simulink model "inv_rot_pen_simscape_vs_analytical_vs_detailed_sim_vs_real"  (R2025b)
settings: Solver=FixedStepAuto  StartTime=0.0  StopTime=4  FixedStep=Ts_fast  MaxStep=1e-3  RelTol=1e-3
values from neighbouring files (symbols this model uses):
  cfg = loaded.cfg    [continueFurutaMatlabSwingupTraining.m]    (also in evaluateFurutaController.m = makeFurutaConfig(); evaluateFurutaMatlabSwingupAgent.m = makeFurutaMatlabSwingupTD3Config(); finalizeFurutaDirectTD3Run.m = normalizeRunConfig(cfg, runDir); initFurutaSldrtHardwareWorkspace.m = makeFurutaMathWorksStyleWideTD3Config())
  i_max = 4    [initFurutaModelWorkspace.m]
  Kp_i = db2mag(options.CurrentControllerKpDb)    [initFurutaModelWorkspace.m]    (also in initFurutaSldrtHardwareWorkspace.m = 2.5)
  omega0 = options.InitialOmega    [initFurutaModelWorkspace.m]
  param = get_parameter()    [initFurutaModelWorkspace.m]
  s = zpk("s")    [initFurutaModelWorkspace.m]    (also in initFurutaSldrtHardwareWorkspace.m)
  theta0 = options.InitialTheta    [initFurutaModelWorkspace.m]
  Tn_i = param.L / param.R    [initFurutaModelWorkspace.m]    (also in initFurutaSldrtHardwareWorkspace.m = 0.000286849073257)
  Ts_fast = cfg.Model.HardwareFastSampleTime    [initFurutaSldrtHardwareWorkspace.m]
undefined symbols (not defined in the file or in its folder): currentBias_A, currentNoiseStd_A, DiscIntNeverNeededParam, G_diff_theta1_ss, G_diff_theta2, G_diff_theta2_ss, G_encoder_notch_d_ss, X, Y, Z
libraries: sm_lib x57, nesl_utility x18, cstblocks x13
(part 1 of 3)
settings Model: Creator=pichim  LastModifiedBy=abuj

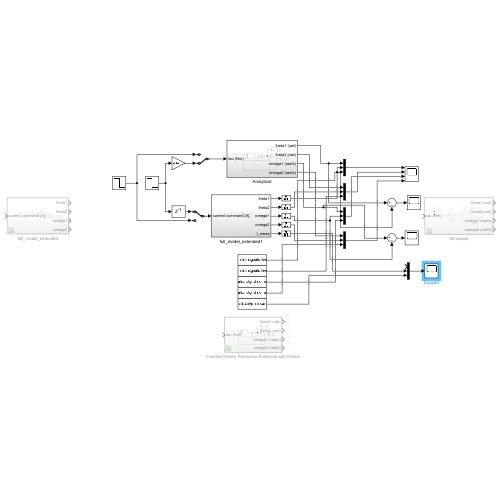
[thumbnail: Simulink's stored preview of the top-level diagram]
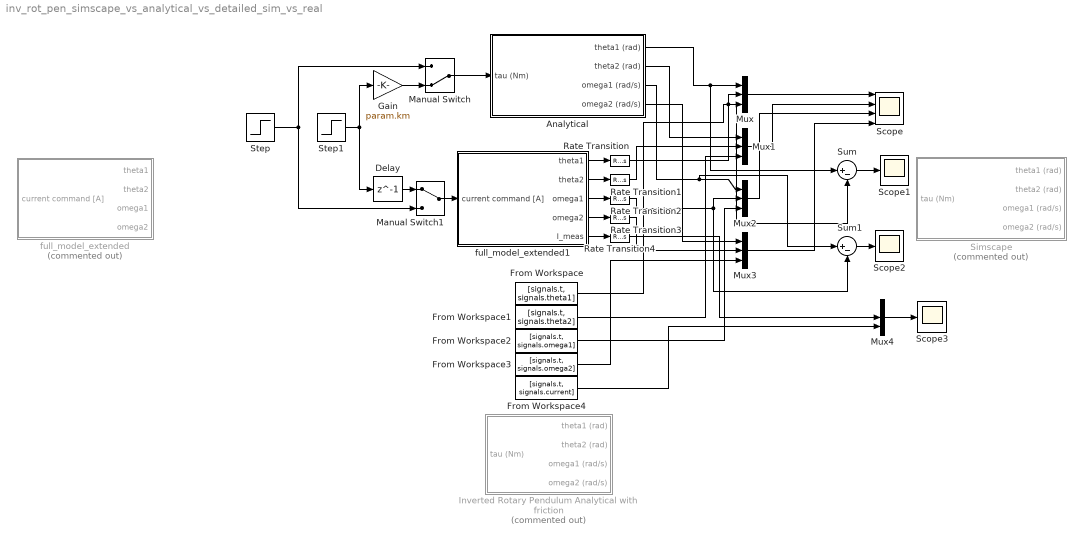
== system inv_rot_pen_simscape_vs_analytical_vs_detailed_sim_vs_real ==
  Analytical : Subsystem
  Delay : Delay  DelayLength=1  SampleTime=1/500
  From Workspace : FromWorkspace  VariableName=[signals.t, signals.theta1]  SampleTime=1/500
  From Workspace1 : FromWorkspace  VariableName=[signals.t, signals.theta2]  SampleTime=1/500
  From Workspace2 : FromWorkspace  VariableName=[signals.t, signals.omega1]  SampleTime=1/500
  From Workspace3 : FromWorkspace  VariableName=[signals.t, signals.omega2]  SampleTime=1/500
  From Workspace4 : FromWorkspace  VariableName=[signals.t, signals.current]  SampleTime=1/500
  Gain : Gain  Gain=param.km
  Inverted Rotary Pendulum Analytical with friction : Subsystem  Commented=on
  Manual Switch : ManualSwitch  CurrentSetting=0
  Manual Switch1 : ManualSwitch
  Mux{,1..4} (5 alike) : Mux  Inputs=3
  Rate Transition{,1..4} (5 alike) : RateTransition
  Scope : Scope  NumInputPorts=4
      settings: ActiveDisplayYMinimum=-12.986747715300275  ActiveDisplayYMaximum=116.88072943770251
  Scope1 : Scope
      settings: ActiveDisplayYMinimum=-1  ActiveDisplayYMaximum=1
  Scope2 : Scope
      settings: ActiveDisplayYMinimum=-2.0883433193053991  ActiveDisplayYMaximum=11.398077430675681
  Scope3 : Scope
      settings: ActiveDisplayYMinimum=-0.11438971016722502  ActiveDisplayYMaximum=0.40266044127837297  DataLoggingVariableName=ScopeData7
  Simscape : Subsystem  Commented=on
  Step : Step  Time=1e-3  Before=10  After=0  SampleTime=0
  Step1 : Step  Time=0.8  Before=0.2  After=0  SampleTime=0
  Sum : Sum  Inputs=|+-
  Sum1 : Sum  Inputs=|+-
  full_model_extended : Subsystem  Commented=on
  full_model_extended1 : Subsystem
  wires:
  Analytical/1(theta1 (rad)) -> Sum/1, Mux/1
  full_model_extended1/1(theta1) -> Rate Transition/1
  Analytical/2(theta2 (rad)) -> Mux1/1
  Rate Transition1/1 -> Mux1/2
  Analytical/3(omega1 (rad/s)) -> Sum1/1, Mux2/1
  Rate Transition2/1 -> Sum1/2, Mux2/2
  Analytical/4(omega2 (rad/s)) -> Mux3/1
  Rate Transition3/1 -> Mux3/2
  Mux/1 -> Scope/1
  Mux1/1 -> Scope/2
  Mux2/1 -> Scope/3
  Mux3/1 -> Scope/4
  Sum/1 -> Scope1/1
  Sum1/1 -> Scope2/1
  Manual Switch1/1 -> full_model_extended1/1(current command [A])
  Manual Switch/1 -> Analytical/1(tau (Nm))
  Step/1 -> Manual Switch1/2, Manual Switch/1
  Gain/1 -> Manual Switch/2
  Step1/1 -> Delay/1, Gain/1
  From Workspace/1 -> Mux/3
  From Workspace3/1 -> Mux3/3
  From Workspace2/1 -> Mux2/3
  From Workspace1/1 -> Mux1/3
  Delay/1 -> Manual Switch1/1
  Rate Transition4/1 -> Mux4/2
  From Workspace4/1 -> Mux4/3
  Mux4/1 -> Scope3/1
  Rate Transition/1 -> Sum/2, Mux/2
  full_model_extended1/3(omega1) -> Rate Transition2/1
  full_model_extended1/2(theta2) -> Rate Transition1/1
  full_model_extended1/4(omega2) -> Rate Transition3/1
  full_model_extended1/5(I_meas) -> Rate Transition4/1

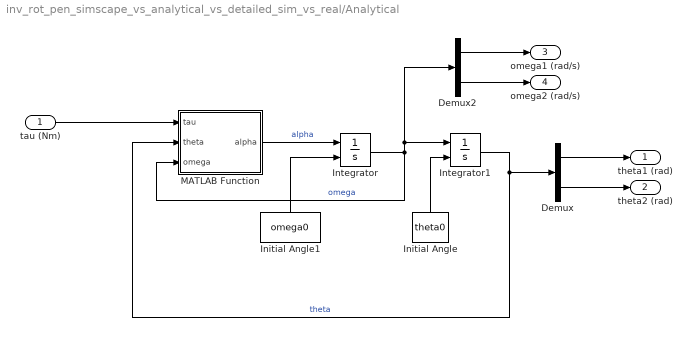
== system inv_rot_pen_simscape_vs_analytical_vs_detailed_sim_vs_real/Analytical ==
  tau (Nm) : Inport
  Demux : Demux  Outputs=2
  Demux2 : Demux  Outputs=2
  Initial Angle : Constant  Value=theta0
  Initial Angle1 : Constant  Value=omega0
  Integrator : Integrator  InitialConditionSource=external
  Integrator1 : Integrator  InitialConditionSource=external  InitialCondition=[0.1;0]
  MATLAB Function : MATLAB Function  TreatAsAtomicUnit=on
  theta1 (rad) : Outport
  theta2 (rad) : Outport  Port=2
  omega1 (rad/s) : Outport  Port=3
  omega2 (rad/s) : Outport  Port=4
  wires:
  Demux/2 -> theta2 (rad)/1
  MATLAB Function/1(alpha) -> Integrator/1  "alpha"
  tau (Nm)/1 -> MATLAB Function/1(tau)
  Integrator1/1 -> MATLAB Function/2(theta), Demux/1  "theta"
  Demux/1 -> theta1 (rad)/1
  Integrator/1 -> Demux2/1, Integrator1/1, MATLAB Function/3(omega)  "omega"
  Demux2/1 -> omega1 (rad/s)/1
  Initial Angle/1 -> Integrator1/2
  Demux2/2 -> omega2 (rad/s)/1
  Initial Angle1/1 -> Integrator/2

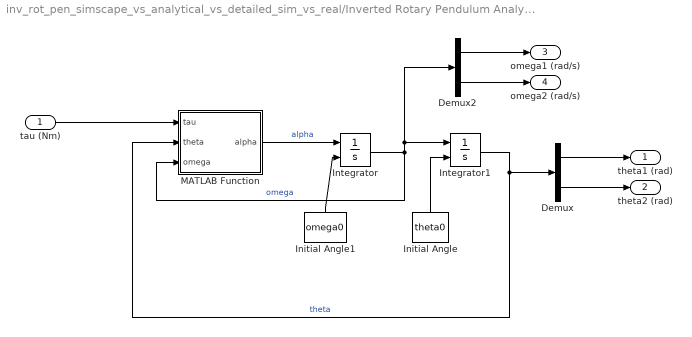
== system inv_rot_pen_simscape_vs_analytical_vs_detailed_sim_vs_real/Inverted Rotary Pendulum Analytical with friction ==
  tau (Nm) : Inport
  Demux : Demux  Outputs=2
  Demux2 : Demux  Outputs=2
  Initial Angle : Constant  Value=theta0
  Initial Angle1 : Constant  Value=omega0
  Integrator : Integrator  InitialConditionSource=external
  Integrator1 : Integrator  InitialConditionSource=external  InitialCondition=[0.1;0]
  MATLAB Function : MATLAB Function  TreatAsAtomicUnit=on
  theta1 (rad) : Outport
  theta2 (rad) : Outport  Port=2
  omega1 (rad/s) : Outport  Port=3
  omega2 (rad/s) : Outport  Port=4
  wires:
  Initial Angle1/1 -> Integrator/2
  Demux2/2 -> omega2 (rad/s)/1
  Initial Angle/1 -> Integrator1/2
  Demux2/1 -> omega1 (rad/s)/1
  Integrator/1 -> MATLAB Function/3(omega), Integrator1/1, Demux2/1  "omega"
  Demux/1 -> theta1 (rad)/1
  Integrator1/1 -> Demux/1, MATLAB Function/2(theta)  "theta"
  tau (Nm)/1 -> MATLAB Function/1(tau)
  MATLAB Function/1(alpha) -> Integrator/1  "alpha"
  Demux/2 -> theta2 (rad)/1

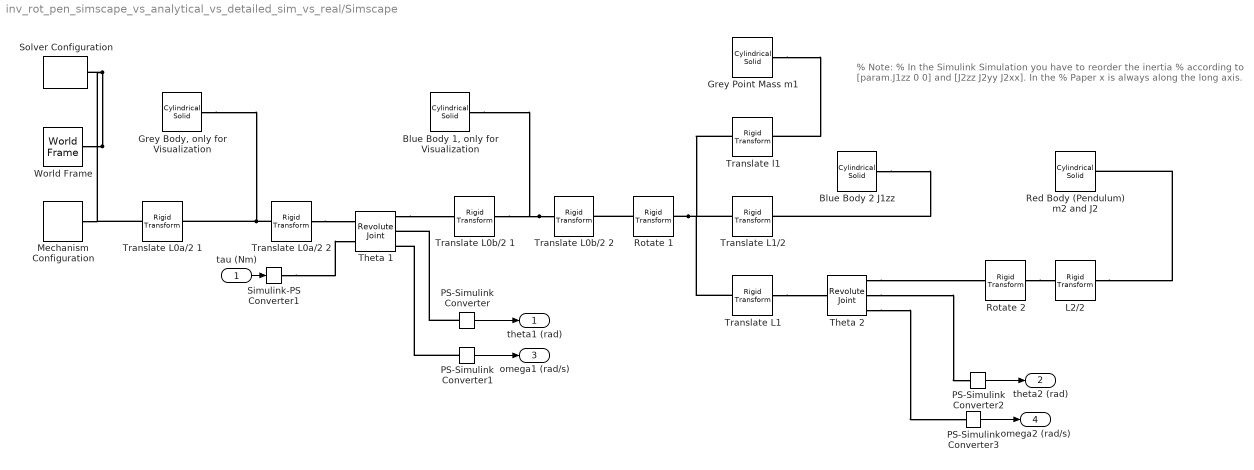
== system inv_rot_pen_simscape_vs_analytical_vs_detailed_sim_vs_real/Simscape ==
  note: % Note:
      | % In the Simulink Simulation you have to reorder the inertia
      | % according to [param.J1zz 0 0] and [J2zz J2yy J2xx]. In the
      | % Paper x is always along the long axis.
  tau (Nm) : Inport
  "Blue Body 1, only for Visualization" : sm_lib/Body Elements/Cylindrical Solid  CylinderRadius=param.r0b  CylinderRadiusUnits=m  CylinderLength=param.L0b  CylinderLengthUnits=m  ExportEntireGeometry=off  InertiaType=PointMass  BasedOnType=Density  Density=1000  DensityUnits=kg/m^3  Mass=0  MassUnits=kg  CenterOfMass=[0 0 0]  CenterOfMassUnits=m  MomentsOfInertia=[0 0 0]  MomentsOfInertiaUnits=kg*m^2  ProductsOfInertia=[0 0 0]  ProductsOfInertiaUnits=kg*m^2  GraphicType=FromGeometry  MarkerShape=Sphere  MarkerSize=10  GraphicVisPropType=SimpleVisualProperties  GraphicDiffuseColor=[0.0 0.6 1.0]  GraphicOpacity=1  GraphicSpecularColor=[0.5 0.5 0.5 1.0]  GraphicAmbientColor=[0.15 0.15 0.15 1.0]  GraphicEmissiveColor=[0.0 0.0 0.0 1.0]  GraphicShininess=75  DoExposeReferenceFrame=on  SerializedFrames=<Frames/>
  Blue Body 2 J1zz : sm_lib/Body Elements/Cylindrical Solid  CylinderRadius=param.r1  CylinderRadiusUnits=m  CylinderLength=param.L1  CylinderLengthUnits=m  ExportEntireGeometry=off  InertiaType=Custom  BasedOnType=Density  Density=1000  DensityUnits=kg/m^3  Mass=0  MassUnits=kg  CenterOfMass=[0 0 0]  CenterOfMassUnits=m  MomentsOfInertia=[param.J1zz 0 0]  MomentsOfInertiaUnits=kg*m^2  ProductsOfInertia=[0 0 0]  ProductsOfInertiaUnits=kg*m^2  GraphicType=FromGeometry  MarkerShape=Sphere  MarkerSize=10  GraphicVisPropType=SimpleVisualProperties  GraphicDiffuseColor=[0.0 0.6 1.0]  GraphicOpacity=1  GraphicSpecularColor=[0.5 0.5 0.5 1.0]  GraphicAmbientColor=[0.15 0.15 0.15 1.0]  GraphicEmissiveColor=[0.0 0.0 0.0 1.0]  GraphicShininess=75  DoExposeReferenceFrame=on  SerializedFrames=<Frames/>
  "Grey Body, only for Visualization" : sm_lib/Body Elements/Cylindrical Solid  CylinderRadius=param.r0a  CylinderRadiusUnits=m  CylinderLength=param.L0a  CylinderLengthUnits=m  ExportEntireGeometry=off  InertiaType=PointMass  BasedOnType=Density  Density=1000  DensityUnits=kg/m^3  Mass=0  MassUnits=kg  CenterOfMass=[0 0 0]  CenterOfMassUnits=m  MomentsOfInertia=[0 0 0]  MomentsOfInertiaUnits=kg*m^2  ProductsOfInertia=[0 0 0]  ProductsOfInertiaUnits=kg*m^2  GraphicType=FromGeometry  MarkerShape=Sphere  MarkerSize=10  GraphicVisPropType=SimpleVisualProperties  GraphicDiffuseColor=[0.5 0.5 0.5]  GraphicOpacity=1  GraphicSpecularColor=[0.5 0.5 0.5 1.0]  GraphicAmbientColor=[0.15 0.15 0.15 1.0]  GraphicEmissiveColor=[0.0 0.0 0.0 1.0]  GraphicShininess=75  DoExposeReferenceFrame=on  SerializedFrames=<Frames/>
  Grey Point Mass m1 : sm_lib/Body Elements/Cylindrical Solid  CylinderRadius=1  CylinderRadiusUnits=m  CylinderLength=1  CylinderLengthUnits=m  ExportEntireGeometry=off  InertiaType=PointMass  BasedOnType=Density  Density=1000  DensityUnits=kg/m^3  Mass=param.m1  MassUnits=kg  CenterOfMass=[0 0 0]  CenterOfMassUnits=m  MomentsOfInertia=[1 1 1]  MomentsOfInertiaUnits=kg*m^2  ProductsOfInertia=[0 0 0]  ProductsOfInertiaUnits=kg*m^2  GraphicType=Marker  MarkerShape=Sphere  MarkerSize=10  GraphicVisPropType=SimpleVisualProperties  GraphicDiffuseColor=[0.5 0.5 0.5]  GraphicOpacity=1  GraphicSpecularColor=[0.5 0.5 0.5 1.0]  GraphicAmbientColor=[0.15 0.15 0.15 1.0]  GraphicEmissiveColor=[0.0 0.0 0.0 1.0]  GraphicShininess=75  DoExposeReferenceFrame=on  SerializedFrames=<Frames/>
  L2/2 : sm_lib/Frames and Transforms/Rigid Transform  RotationMethod=None  FollAlignAxisA=+X  BaseAlignAxisA=+Y  FollAlignAxisB=+Y  BaseAlignAxisB=+Z  RotationStandardAxis=+Z  RotationAngle=0  RotationAngleUnits=deg  RotationArbitraryAxis=[0 0 1]  RotationSequenceAxes=FollowerAxes  RotationSequence=ZYX  RotationSequenceAngles=[0 pi/2 0]  RotationSequenceAnglesUnits=rad  RotationMatrix=[1 0 0;0 1 0;0 0 1]  Quaternion=[1 0 0 0]  TranslationMethod=Cartesian  TranslationCartesianOffset=[0 0 param.L2/2]  TranslationCartesianOffsetUnits=m  TranslationStandardAxis=+Z  TranslationStandardOffset=0  TranslationStandardOffsetUnits=m  TranslationROffset=0  TranslationROffsetUnits=m  TranslationThetaOffset=0  TranslationThetaOffsetUnits=deg  TranslationZOffset=0  TranslationZOffsetUnits=m
  Mechanism Configuration : sm_lib/Utilities/Mechanism Configuration  UniformGravity=Constant  GravityVector=[0 0 -param.g]  GravityVectorUnits=m/s^2  LinearizationDelta=0.001  JointModeTransitionNonlinearIterations=2
  PS-Simulink Converter{,1..3} (4 alike) : nesl_utility/PS-Simulink Converter  PhysicalDomain=network_engine_domain  SubClassName=ps_output  LeftPortType=input  RightPortType=output  PseudoPeriodic=off  Frequencies=[]  VectorFormat=inherit  Unit=inherit  AffineConversion=off
  Red Body (Pendulum) m2 and J2 : sm_lib/Body Elements/Cylindrical Solid  CylinderRadius=param.r2  CylinderRadiusUnits=m  CylinderLength=param.L2  CylinderLengthUnits=m  ExportEntireGeometry=off  InertiaType=Custom  BasedOnType=Density  Density=1000  DensityUnits=kg/m^3  Mass=param.m2  MassUnits=kg  CenterOfMass=[0 0 0]  CenterOfMassUnits=m  MomentsOfInertia=[param.J2zz param.J2yy param.J2xx]  MomentsOfInertiaUnits=kg*m^2  ProductsOfInertia=[0 0 0]  ProductsOfInertiaUnits=kg*m^2  GraphicType=FromGeometry  MarkerShape=Sphere  MarkerSize=10  GraphicVisPropType=SimpleVisualProperties  GraphicDiffuseColor=[1.0 0.2 0.2]  GraphicOpacity=1  GraphicSpecularColor=[0.5 0.5 0.5 1.0]  GraphicAmbientColor=[0.15 0.15 0.15 1.0]  GraphicEmissiveColor=[0.0 0.0 0.0 1.0]  GraphicShininess=75  DoExposeReferenceFrame=on  SerializedFrames=<Frames/>
  Rotate 1 : sm_lib/Frames and Transforms/Rigid Transform  RotationMethod=RotationSequence  FollAlignAxisA=+X  BaseAlignAxisA=+Y  FollAlignAxisB=+Y  BaseAlignAxisB=+Z  RotationStandardAxis=+Z  RotationAngle=0  RotationAngleUnits=deg  RotationArbitraryAxis=[0 0 1]  RotationSequenceAxes=FollowerAxes  RotationSequence=ZYX  RotationSequenceAngles=[0 pi/2 0]  RotationSequenceAnglesUnits=rad  RotationMatrix=[1 0 0;0 1 0;0 0 1]  Quaternion=[1 0 0 0]  TranslationMethod=None  TranslationCartesianOffset=[0 0 0]  TranslationCartesianOffsetUnits=m  TranslationStandardAxis=+Z  TranslationStandardOffset=0  TranslationStandardOffsetUnits=m  TranslationROffset=0  TranslationROffsetUnits=m  TranslationThetaOffset=0  TranslationThetaOffsetUnits=deg  TranslationZOffset=0  TranslationZOffsetUnits=m
  Rotate 2 : sm_lib/Frames and Transforms/Rigid Transform  RotationMethod=RotationSequence  FollAlignAxisA=+X  BaseAlignAxisA=+Y  FollAlignAxisB=+Y  BaseAlignAxisB=+Z  RotationStandardAxis=+Z  RotationAngle=0  RotationAngleUnits=deg  RotationArbitraryAxis=[0 0 1]  RotationSequenceAxes=FollowerAxes  RotationSequence=ZYX  RotationSequenceAngles=[0 pi/2 0]  RotationSequenceAnglesUnits=rad  RotationMatrix=[1 0 0;0 1 0;0 0 1]  Quaternion=[1 0 0 0]  TranslationMethod=None  TranslationCartesianOffset=[0 0 0]  TranslationCartesianOffsetUnits=m  TranslationStandardAxis=+Z  TranslationStandardOffset=0  TranslationStandardOffsetUnits=m  TranslationROffset=0  TranslationROffsetUnits=m  TranslationThetaOffset=0  TranslationThetaOffsetUnits=deg  TranslationZOffset=0  TranslationZOffsetUnits=m
  Simulink-PS Converter1 : nesl_utility/Simulink-PS Converter  PhysicalDomain=network_engine_domain  SubClassName=ps_input  LeftPortType=input  RightPortType=output  PseudoPeriodic=off  Frequencies=[]  NoiseDistribution=none  NoiseParameters=[]  Unit=1  AffineConversion=off  FilteringAndDerivatives=provide  SimscapeFilterOrder=1  InputFilterTimeConstant=0.001  UdotUserProvided=0
  Solver Configuration : nesl_utility/Solver Configuration  PhysicalDomain=network_engine_domain  SubClassName=solver  LeftPortType=input  RightPortType=generic  Tones=[]  Harmonics=[]  SimulateNoise=off  Profile=off  UseLocalSampling=off  EnableSwitchedLinearOptims=on  FrequencyDomain=off  UseCCode=off  RelTol=0.001  AbsTol=0.001  MinStep=1e-09  ToWorkspace=off  RevertToSquareIcSolve=off  NumHomotopyIterations=100  PhasorMode=off  PhasorModeNumHarmonics=1  ConsistencySolver=NEWTON_XTOL_AFTER_FTOL  IndexReductionMethod=DerivativeReplacement  DoDC=off  ResidualTolerance=1e-09  ConsistencyTolSource=GLOBAL  ConsistencyAbsTol=0.001  ConsistencyRelTol=0.001  ConsistencyTolFactor=0.001  UseLocalSolver=off  LocalSolverChoice=NE_BACKWARD_EULER_ADVANCER  ResolveIndetEquations=on  FunctionEvalNumThread=1  LocalSolverSampleTime=0.001  DoFixedCost=off  MaxNonlinIter=3  MaxModeIter=2  ComputeImpulses=off  ImpulseIterations=2  LinearAlgebra=auto  LinearAlgebraNumThread=0  EquationFormulation=NE_TIME_EF  DelaysMemoryBudget=1024  AutomaticFiltering=on  FilteringTimeConstant=0.001  PartitionStorageMethod=AS_NEEDED  PartitionMemoryBudget=1024  PartitionMethod=ROBUST  MultibodyUseLocalSolver=off  MultibodyLocalSolverChoice=ODE1  MultibodyLocalSolverSampleTime=0.001
  Theta 1 : sm_lib/Joints/Revolute Joint  JointMode=Normal  CompositeWrenchDir=FollowerOnBase  CompositeWrenchFrame=BaseFrame  SenseConstraintForce=off  SenseConstraintTorque=off  SenseTotalForce=off  SenseTotalTorque=off  PositionTargetSpecify=on  PositionTargetPriority=High  PositionTargetValue=theta0(1)  PositionTargetValueUnits=rad  VelocityTargetSpecify=off  VelocityTargetPriority=High  VelocityTargetValue=0  VelocityTargetValueUnits=deg/s  EquilibriumPosition=0  EquilibriumPositionUnits=rad  SpringStiffness=0  SpringStiffnessUnits=N*m/rad  DampingCoefficient=param.b1  DampingCoefficientUnits=N*m*s/rad  LowerLimitSpecify=off  LowerLimitBound=-90  LowerLimitBoundUnits=deg  LowerLimitStiffness=1e4  LowerLimitStiffnessUnits=N*m/deg  LowerLimitDamping=10  LowerLimitDampingUnits=N*m/(deg/s)  LowerLimitTransitionRegionWidth=0.1  LowerLimitTransitionRegionWidthUnits=deg  UpperLimitSpecify=off  UpperLimitBound=90  UpperLimitBoundUnits=deg  UpperLimitStiffness=1e4  UpperLimitStiffnessUnits=N*m/deg  UpperLimitDamping=10  UpperLimitDampingUnits=N*m/(deg/s)  UpperLimitTransitionRegionWidth=0.1  UpperLimitTransitionRegionWidthUnits=deg  TorqueActuationMode=InputTorque  MotionActuationMode=ComputedMotion  SensePosition=on  SenseVelocity=on  SenseAcceleration=off  SenseTorqueForce=off  SenseLowerLimitTorqueForce=off  SenseUpperLimitTorqueForce=off
  Theta 2 : sm_lib/Joints/Revolute Joint  JointMode=Normal  CompositeWrenchDir=FollowerOnBase  CompositeWrenchFrame=BaseFrame  SenseConstraintForce=off  SenseConstraintTorque=off  SenseTotalForce=off  SenseTotalTorque=off  PositionTargetSpecify=on  PositionTargetPriority=High  PositionTargetValue=theta0(2)  PositionTargetValueUnits=rad  VelocityTargetSpecify=off  VelocityTargetPriority=High  VelocityTargetValue=0  VelocityTargetValueUnits=deg/s  EquilibriumPosition=0  EquilibriumPositionUnits=rad  SpringStiffness=0  SpringStiffnessUnits=N*m/rad  DampingCoefficient=param.b2  DampingCoefficientUnits=N*m*s/rad  LowerLimitSpecify=off  LowerLimitBound=-90  LowerLimitBoundUnits=deg  LowerLimitStiffness=1e4  LowerLimitStiffnessUnits=N*m/deg  LowerLimitDamping=10  LowerLimitDampingUnits=N*m/(deg/s)  LowerLimitTransitionRegionWidth=0.1  LowerLimitTransitionRegionWidthUnits=deg  UpperLimitSpecify=off  UpperLimitBound=90  UpperLimitBoundUnits=deg  UpperLimitStiffness=1e4  UpperLimitStiffnessUnits=N*m/deg  UpperLimitDamping=10  UpperLimitDampingUnits=N*m/(deg/s)  UpperLimitTransitionRegionWidth=0.1  UpperLimitTransitionRegionWidthUnits=deg  TorqueActuationMode=NoTorque  MotionActuationMode=ComputedMotion  SensePosition=on  SenseVelocity=on  SenseAcceleration=off  SenseTorqueForce=off  SenseLowerLimitTorqueForce=off  SenseUpperLimitTorqueForce=off
  Translate L0a/2 1 : sm_lib/Frames and Transforms/Rigid Transform  RotationMethod=None  FollAlignAxisA=+X  BaseAlignAxisA=+Y  FollAlignAxisB=+Y  BaseAlignAxisB=+Z  RotationStandardAxis=+Z  RotationAngle=0  RotationAngleUnits=deg  RotationArbitraryAxis=[0 0 1]  RotationSequenceAxes=FollowerAxes  RotationSequence=ZYX  RotationSequenceAngles=[0 0 0]  RotationSequenceAnglesUnits=rad  RotationMatrix=[1 0 0;0 1 0;0 0 1]  Quaternion=[1 0 0 0]  TranslationMethod=Cartesian  TranslationCartesianOffset=[0 0 param.L0a/2]  TranslationCartesianOffsetUnits=m  TranslationStandardAxis=+Z  TranslationStandardOffset=0  TranslationStandardOffsetUnits=m  TranslationROffset=0  TranslationROffsetUnits=m  TranslationThetaOffset=0  TranslationThetaOffsetUnits=deg  TranslationZOffset=0  TranslationZOffsetUnits=m
  Translate L0a/2 2 : sm_lib/Frames and Transforms/Rigid Transform  RotationMethod=None  FollAlignAxisA=+X  BaseAlignAxisA=+Y  FollAlignAxisB=+Y  BaseAlignAxisB=+Z  RotationStandardAxis=+Z  RotationAngle=0  RotationAngleUnits=deg  RotationArbitraryAxis=[0 0 1]  RotationSequenceAxes=FollowerAxes  RotationSequence=ZYX  RotationSequenceAngles=[0 0 0]  RotationSequenceAnglesUnits=rad  RotationMatrix=[1 0 0;0 1 0;0 0 1]  Quaternion=[1 0 0 0]  TranslationMethod=Cartesian  TranslationCartesianOffset=[0 0 param.L0a/2]  TranslationCartesianOffsetUnits=m  TranslationStandardAxis=+Z  TranslationStandardOffset=0  TranslationStandardOffsetUnits=m  TranslationROffset=0  TranslationROffsetUnits=m  TranslationThetaOffset=0  TranslationThetaOffsetUnits=deg  TranslationZOffset=0  TranslationZOffsetUnits=m
  Translate L0b/2 1 : sm_lib/Frames and Transforms/Rigid Transform  RotationMethod=None  FollAlignAxisA=+X  BaseAlignAxisA=+Y  FollAlignAxisB=+Y  BaseAlignAxisB=+Z  RotationStandardAxis=+Z  RotationAngle=0  RotationAngleUnits=deg  RotationArbitraryAxis=[0 0 1]  RotationSequenceAxes=FollowerAxes  RotationSequence=ZYX  RotationSequenceAngles=[0 0 0]  RotationSequenceAnglesUnits=rad  RotationMatrix=[1 0 0;0 1 0;0 0 1]  Quaternion=[1 0 0 0]  TranslationMethod=Cartesian  TranslationCartesianOffset=[0 0 param.L0b/2]  TranslationCartesianOffsetUnits=m  TranslationStandardAxis=+Z  TranslationStandardOffset=0  TranslationStandardOffsetUnits=m  TranslationROffset=0  TranslationROffsetUnits=m  TranslationThetaOffset=0  TranslationThetaOffsetUnits=deg  TranslationZOffset=0  TranslationZOffsetUnits=m
  Translate L0b/2 2 : sm_lib/Frames and Transforms/Rigid Transform  RotationMethod=None  FollAlignAxisA=+X  BaseAlignAxisA=+Y  FollAlignAxisB=+Y  BaseAlignAxisB=+Z  RotationStandardAxis=+Z  RotationAngle=0  RotationAngleUnits=deg  RotationArbitraryAxis=[0 0 1]  RotationSequenceAxes=FollowerAxes  RotationSequence=ZYX  RotationSequenceAngles=[0 0 0]  RotationSequenceAnglesUnits=rad  RotationMatrix=[1 0 0;0 1 0;0 0 1]  Quaternion=[1 0 0 0]  TranslationMethod=Cartesian  TranslationCartesianOffset=[0 0 param.L0b/2]  TranslationCartesianOffsetUnits=m  TranslationStandardAxis=+Z  TranslationStandardOffset=0  TranslationStandardOffsetUnits=m  TranslationROffset=0  TranslationROffsetUnits=m  TranslationThetaOffset=0  TranslationThetaOffsetUnits=deg  TranslationZOffset=0  TranslationZOffsetUnits=m
  Translate L1 : sm_lib/Frames and Transforms/Rigid Transform  RotationMethod=None  FollAlignAxisA=+X  BaseAlignAxisA=+Y  FollAlignAxisB=+Y  BaseAlignAxisB=+Z  RotationStandardAxis=+Z  RotationAngle=0  RotationAngleUnits=deg  RotationArbitraryAxis=[0 0 1]  RotationSequenceAxes=FollowerAxes  RotationSequence=ZYX  RotationSequenceAngles=[0 0 0]  RotationSequenceAnglesUnits=rad  RotationMatrix=[1 0 0;0 1 0;0 0 1]  Quaternion=[1 0 0 0]  TranslationMethod=Cartesian  TranslationCartesianOffset=[0 0 param.L1]  TranslationCartesianOffsetUnits=m  TranslationStandardAxis=+Z  TranslationStandardOffset=0  TranslationStandardOffsetUnits=m  TranslationROffset=0  TranslationROffsetUnits=m  TranslationThetaOffset=0  TranslationThetaOffsetUnits=deg  TranslationZOffset=0  TranslationZOffsetUnits=m
  Translate L1/2 : sm_lib/Frames and Transforms/Rigid Transform  RotationMethod=None  FollAlignAxisA=+X  BaseAlignAxisA=+Y  FollAlignAxisB=+Y  BaseAlignAxisB=+Z  RotationStandardAxis=+Z  RotationAngle=0  RotationAngleUnits=deg  RotationArbitraryAxis=[0 0 1]  RotationSequenceAxes=FollowerAxes  RotationSequence=ZYX  RotationSequenceAngles=[0 0 0]  RotationSequenceAnglesUnits=rad  RotationMatrix=[1 0 0;0 1 0;0 0 1]  Quaternion=[1 0 0 0]  TranslationMethod=Cartesian  TranslationCartesianOffset=[0 0 param.L1/2]  TranslationCartesianOffsetUnits=m  TranslationStandardAxis=+Z  TranslationStandardOffset=0  TranslationStandardOffsetUnits=m  TranslationROffset=0  TranslationROffsetUnits=m  TranslationThetaOffset=0  TranslationThetaOffsetUnits=deg  TranslationZOffset=0  TranslationZOffsetUnits=m
  Translate l1 : sm_lib/Frames and Transforms/Rigid Transform  RotationMethod=None  FollAlignAxisA=+X  BaseAlignAxisA=+Y  FollAlignAxisB=+Y  BaseAlignAxisB=+Z  RotationStandardAxis=+Z  RotationAngle=0  RotationAngleUnits=deg  RotationArbitraryAxis=[0 0 1]  RotationSequenceAxes=FollowerAxes  RotationSequence=ZYX  RotationSequenceAngles=[0 0 0]  RotationSequenceAnglesUnits=rad  RotationMatrix=[1 0 0;0 1 0;0 0 1]  Quaternion=[1 0 0 0]  TranslationMethod=Cartesian  TranslationCartesianOffset=[0 0 param.l1]  TranslationCartesianOffsetUnits=m  TranslationStandardAxis=+Z  TranslationStandardOffset=0  TranslationStandardOffsetUnits=m  TranslationROffset=0  TranslationROffsetUnits=m  TranslationThetaOffset=0  TranslationThetaOffsetUnits=deg  TranslationZOffset=0  TranslationZOffsetUnits=m
  World Frame : sm_lib/Frames and Transforms/World Frame
  theta1 (rad) : Outport
  theta2 (rad) : Outport  Port=2
  omega1 (rad/s) : Outport  Port=3
  omega2 (rad/s) : Outport  Port=4
  wires:
  PS-Simulink Converter3/1 -> omega2 (rad/s)/1
  PS-Simulink Converter2/1 -> theta2 (rad)/1
  PS-Simulink Converter/1 -> theta1 (rad)/1
  PS-Simulink Converter1/1 -> omega1 (rad/s)/1
  tau (Nm)/1 -> Simulink-PS Converter1/1
  connections:
  Solver Configuration/RConn1 -- Translate L0a/2 1/LConn1 -- Mechanism Configuration/RConn1 -- World Frame/RConn1
  Translate L0b/2 2/LConn1 -- "Blue Body 1, only for Visualization"/RConn1 -- Translate L0b/2 1/RConn1
  Translate L0a/2 2/LConn1 -- "Grey Body, only for Visualization"/RConn1 -- Translate L0a/2 1/RConn1
  Rotate 1/RConn1 -- Translate L1/2/LConn1 -- Translate L1/LConn1 -- Translate l1/LConn1
  Rotate 1/LConn1 -- Translate L0b/2 2/RConn1
  Theta 2/RConn3 -- PS-Simulink Converter3/LConn1
  L2/2/RConn1 -- Red Body (Pendulum) m2 and J2/RConn1
  Theta 1/RConn1 -- Translate L0b/2 1/LConn1
  Theta 2/RConn2 -- PS-Simulink Converter2/LConn1
  Theta 2/RConn1 -- Rotate 2/LConn1
  Blue Body 2 J1zz/RConn1 -- Translate L1/2/RConn1
  Grey Point Mass m1/RConn1 -- Translate l1/RConn1
  Translate L1/RConn1 -- Theta 2/LConn1
  Rotate 2/RConn1 -- L2/2/LConn1
  Translate L0a/2 2/RConn1 -- Theta 1/LConn1
  PS-Simulink Converter1/LConn1 -- Theta 1/RConn3
  PS-Simulink Converter/LConn1 -- Theta 1/RConn2
  Simulink-PS Converter1/RConn1 -- Theta 1/LConn2

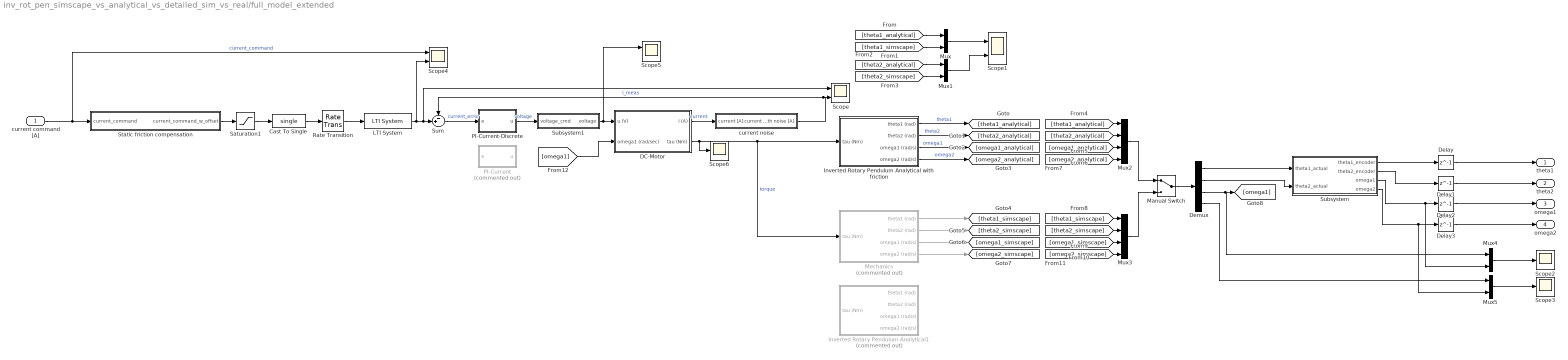
== system inv_rot_pen_simscape_vs_analytical_vs_detailed_sim_vs_real/full_model_extended ==
  current command [A] : Inport
  Cast To Single : DataTypeConversion  OutDataTypeStr=single  SaturateOnIntegerOverflow=off  RndMeth=Floor
  DC-Motor : Subsystem
  Delay{,1..3} (4 alike) : Delay  DelayLength=1  SampleTime=1/500
  Demux : Demux
  Inverted Rotary Pendulum Analytical with friction : Subsystem
  Inverted Rotary Pendulum Analytical1 : Subsystem  Commented=on
  LTI System : cstblocks/LTI System  sys=G_i_cmd_lpf_d  IC=[]  PadeOrder=0
  Manual Switch : ManualSwitch
  Mechanics : Subsystem  Commented=on
  Mux{,1,4..5} (4 alike) : Mux  Inputs=2
  Mux2 : Mux
  Mux3 : Mux
  PI-Current : Subsystem  Commented=on
  PI-Current-Discrete : Subsystem
  Rate Transition : RateTransition  OutPortSampleTime=Ts_fast
  Saturation1 : Saturate  UpperLimit=i_max  LowerLimit=-i_max
  Scope{,1,4..5} (4 alike) : Scope  NumInputPorts=2
      Scope settings: ActiveDisplayYMinimum=-0.19954742270611825  ActiveDisplayYMaximum=0.40065017446968165
      Scope1 settings: ActiveDisplayYMinimum=-1.8621582000632775  ActiveDisplayYMaximum=1.0563365896676562  DataLoggingVariableName=ScopeData6
      Scope4 settings: ActiveDisplayYMinimum=-1.2561628236435352  ActiveDisplayYMaximum=11.250684758182615  DataLoggingVariableName=ScopeData2
      Scope5 settings: ActiveDisplayYMinimum=-5.2313259780059385  ActiveDisplayYMaximum=27.070147330889547  DataLoggingVariableName=ScopeData4
  Scope2 : Scope
  Scope3 : Scope
      settings: DataLoggingVariableName=ScopeData3
  Scope6 : Scope
      settings: ActiveDisplayYMinimum=-0.050293714673501369  ActiveDisplayYMaximum=0.30475707690688031  DataLoggingVariableName=ScopeData5
  Static friction compensation : Subsystem
  Subsystem : Subsystem
  Subsystem1 : Subsystem
  Sum : Sum  Inputs=-+|
  current noise : Subsystem
  theta1 : Outport
  theta2 : Outport  Port=2
  omega1 : Outport  Port=3
  omega2 : Outport  Port=4
  wires:
  [omega1] -> DC-Motor/2(omega1 (rad/sec))
  Manual Switch/1 -> Demux/1
  Demux/2 -> Subsystem/2(theta2_actual)
  Demux/1 -> Subsystem/1(theta1_actual)
  Mux3/1 -> Manual Switch/2
  [omega2_simscape] -> Mux3/4
  [omega1_simscape] -> Mux3/3
  [theta2_simscape] -> Mux3/2
  [theta1_simscape] -> Mux3/1
  [omega2_analytical] -> Mux2/4
  [omega1_analytical] -> Mux2/3
  [theta2_analytical] -> Mux2/2
  [theta1_analytical] -> Mux2/1
  Mux2/1 -> Manual Switch/1
  [theta2_simscape] -> Mux1/2
  [theta2_analytical] -> Mux1/1
  [theta1_simscape] -> Mux/2
  [theta1_analytical] -> Mux/1
  Mechanics/4(omega2 (rad/s)) -> [omega2_simscape]
  Mechanics/3(omega1 (rad/s)) -> [omega1_simscape]
  Mechanics/2(theta2 (rad)) -> [theta2_simscape]
  Mechanics/1(theta1 (rad)) -> [theta1_simscape]
  Mux1/1 -> Scope1/2
  Mux/1 -> Scope1/1
  Sum/1 -> PI-Current-Discrete/1(e)  "current_error"
  DC-Motor/1(i (A)) -> current noise/1(current [A])  "current"
  DC-Motor/2(tau (Nm)) -> Scope6/1, Inverted Rotary Pendulum Analytical with friction/1(tau (Nm)), Mechanics/1(tau (Nm))  "torque"
  Inverted Rotary Pendulum Analytical with friction/2(theta2 (rad)) -> [theta2_analytical]  "theta2"
  Inverted Rotary Pendulum Analytical with friction/4(omega2 (rad/s)) -> [omega2_analytical]  "omega2"
  Inverted Rotary Pendulum Analytical with friction/1(theta1 (rad)) -> [theta1_analytical]  "theta1"
  Inverted Rotary Pendulum Analytical with friction/3(omega1 (rad/s)) -> [omega1_analytical]  "omega1"
  current noise/1(current with noise [A]) -> Sum/1, Scope/2  "i_meas"
  Saturation1/1 -> Cast To Single/1
  Subsystem/1(theta1_encoder) -> Delay/1
  Subsystem/2(theta2_encoder) -> Delay1/1
  Subsystem/3(omega1) -> Mux4/2, Delay2/1
  Subsystem/4(omega2) -> Mux5/2, Delay3/1
  Mux4/1 -> Scope2/1
  Demux/3 -> Mux4/1, [omega1]
  Mux5/1 -> Scope3/1
  Demux/4 -> Mux5/1
  Cast To Single/1 -> Rate Transition/1
  LTI System/1 -> Scope4/2, Scope/1, Sum/2
  Rate Transition/1 -> LTI System/1
  PI-Current-Discrete/1(u) -> Subsystem1/1(voltage_cmd)  "voltage"
  Subsystem1/1(voltage) -> Scope5/1, DC-Motor/1(u (V))
  current command [A]/1 -> Scope4/1, Static friction compensation/1(current_command)  "current_command"
  Static friction compensation/1(current_command_w_offset) -> Saturation1/1
  Delay/1 -> theta1/1
  Delay1/1 -> theta2/1
  Delay2/1 -> omega1/1
  Delay3/1 -> omega2/1

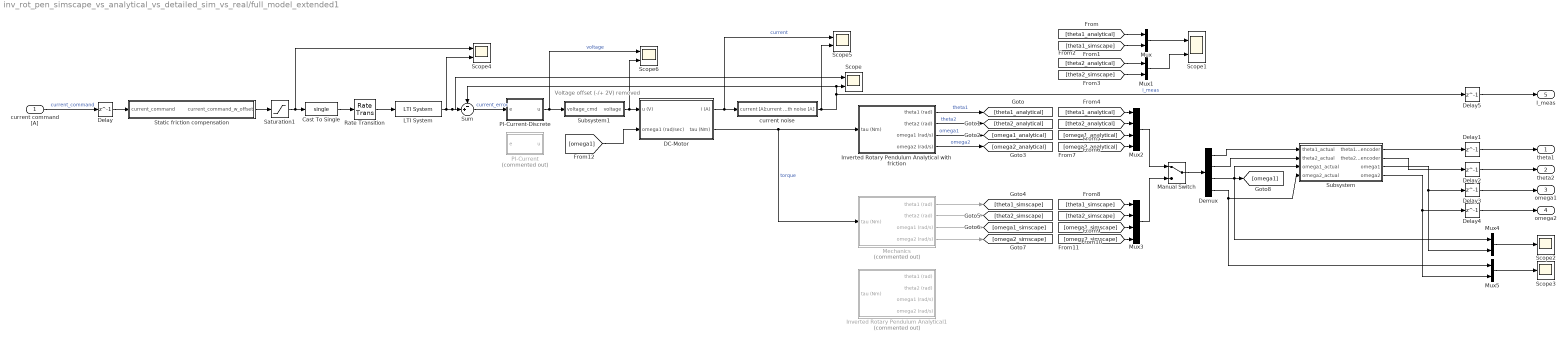
== system inv_rot_pen_simscape_vs_analytical_vs_detailed_sim_vs_real/full_model_extended1 ==
  note: Voltage offset (-/+ 2V) removed
  current command [A] : Inport
  Cast To Single : DataTypeConversion  OutDataTypeStr=single  SaturateOnIntegerOverflow=off  RndMeth=Floor
  DC-Motor : Subsystem
  Delay{,1..5} (6 alike) : Delay  DelayLength=1  SampleTime=cfg.Agent.SampleTime
  Demux : Demux
  Inverted Rotary Pendulum Analytical with friction : Subsystem
  Inverted Rotary Pendulum Analytical1 : Subsystem  Commented=on
  LTI System : cstblocks/LTI System  sys=G_i_cmd_lpf_d  IC=[]  PadeOrder=0
  Manual Switch : ManualSwitch
  Mechanics : Subsystem  Commented=on
  Mux{,1,4..5} (4 alike) : Mux  Inputs=2
  Mux2 : Mux
  Mux3 : Mux
  PI-Current : Subsystem  Commented=on
  PI-Current-Discrete : Subsystem
  Rate Transition : RateTransition  OutPortSampleTime=Ts_fast
  Saturation1 : Saturate  UpperLimit=i_max  LowerLimit=-i_max
  Scope{,1,4..6} (5 alike) : Scope  NumInputPorts=2
      Scope settings: ActiveDisplayYMinimum=-0.69637994539931947  ActiveDisplayYMaximum=0.69318633871495239
      Scope1 settings: ActiveDisplayYMinimum=-1.8621582000632775  ActiveDisplayYMaximum=1.0563365896676562  DataLoggingVariableName=ScopeData6
      Scope4 settings: ActiveDisplayYMinimum=-0.65187358111143112  ActiveDisplayYMaximum=0.65203338116407394  DataLoggingVariableName=ScopeData8
      Scope5 settings: ActiveDisplayYMinimum=-0.046106222305020483  ActiveDisplayYMaximum=0.045330327902423417  DataLoggingVariableName=ScopeData9
      Scope6 settings: ActiveDisplayYMinimum=-0.55228723856993833  ActiveDisplayYMaximum=3.9586657201678768  DataLoggingVariableName=ScopeData10
  Scope2 : Scope
      settings: ActiveDisplayYMinimum=-9.2948883098113519  ActiveDisplayYMaximum=40.102948404182051
  Scope3 : Scope
      settings: ActiveDisplayYMinimum=-24.943568620933455  ActiveDisplayYMaximum=30.626305547679333  DataLoggingVariableName=ScopeData3
  Static friction compensation : Subsystem
  Subsystem : Subsystem
  Subsystem1 : Subsystem
  Sum : Sum  Inputs=-+|
  current noise : Subsystem
  theta1 : Outport
  theta2 : Outport  Port=2
  omega1 : Outport  Port=3
  omega2 : Outport  Port=4
  I_meas : Outport  Port=5
  wires:
  [omega1] -> DC-Motor/2(omega1 (rad/sec))
  Manual Switch/1 -> Demux/1
  Demux/2 -> Subsystem/2(theta2_actual)
  Demux/1 -> Subsystem/1(theta1_actual)
  Mux3/1 -> Manual Switch/2
  [omega2_simscape] -> Mux3/4
  [omega1_simscape] -> Mux3/3
  [theta2_simscape] -> Mux3/2
  [theta1_simscape] -> Mux3/1
  [omega2_analytical] -> Mux2/4
  [omega1_analytical] -> Mux2/3
  [theta2_analytical] -> Mux2/2
  [theta1_analytical] -> Mux2/1
  Mux2/1 -> Manual Switch/1
  [theta2_simscape] -> Mux1/2
  [theta2_analytical] -> Mux1/1
  [theta1_simscape] -> Mux/2
  [theta1_analytical] -> Mux/1
  Mechanics/4(omega2 (rad/s)) -> [omega2_simscape]
  Mechanics/3(omega1 (rad/s)) -> [omega1_simscape]
  Mechanics/2(theta2 (rad)) -> [theta2_simscape]
  Mechanics/1(theta1 (rad)) -> [theta1_simscape]
  Mux1/1 -> Scope1/2
  Mux/1 -> Scope1/1
  Sum/1 -> PI-Current-Discrete/1(e)  "current_error"
  DC-Motor/1(i (A)) -> Scope5/1, current noise/1(current [A])  "current"
  DC-Motor/2(tau (Nm)) -> Inverted Rotary Pendulum Analytical with friction/1(tau (Nm)), Mechanics/1(tau (Nm))  "torque"
  Inverted Rotary Pendulum Analytical with friction/2(theta2 (rad)) -> [theta2_analytical]  "theta2"
  Inverted Rotary Pendulum Analytical with friction/4(omega2 (rad/s)) -> [omega2_analytical]  "omega2"
  Inverted Rotary Pendulum Analytical with friction/1(theta1 (rad)) -> [theta1_analytical]  "theta1"
  Inverted Rotary Pendulum Analytical with friction/3(omega1 (rad/s)) -> [omega1_analytical]  "omega1"
  current noise/1(current with noise [A]) -> Scope5/2, Delay5/1, Sum/1, Scope/2  "i_meas"
  Saturation1/1 -> Scope4/1, Cast To Single/1
  Subsystem/1(theta1_encoder) -> Delay1/1
  Subsystem/2(theta2_encoder) -> Delay2/1
  Subsystem/3(omega1) -> Mux4/2, Delay3/1
  Subsystem/4(omega2) -> Mux5/2, Delay4/1
  Mux4/1 -> Scope2/1
  Demux/3 -> Mux4/1, Subsystem/3(omega1_actual), [omega1]
  Mux5/1 -> Scope3/1
  Demux/4 -> Subsystem/4(omega2_actual), Mux5/1
  Cast To Single/1 -> Rate Transition/1
  LTI System/1 -> Scope4/2, Scope/1, Sum/2
  Rate Transition/1 -> LTI System/1
  PI-Current-Discrete/1(u) -> Scope6/1, Subsystem1/1(voltage_cmd)  "voltage"
  Subsystem1/1(voltage) -> Scope6/2, DC-Motor/1(u (V))
  current command [A]/1 -> Delay/1  "current_command"
  Static friction compensation/1(current_command_w_offset) -> Saturation1/1
  Delay/1 -> Static friction compensation/1(current_command)
  Delay1/1 -> theta1/1
  Delay2/1 -> theta2/1
  Delay3/1 -> omega1/1
  Delay4/1 -> omega2/1
  Delay5/1 -> I_meas/1

== system inv_rot_pen_simscape_vs_analytical_vs_detailed_sim_vs_real/full_model_extended/DC-Motor ==
  u (V) : Inport
  omega1 (rad/sec) : Inport  Port=2
  1/L : Gain  Gain=1/param.L
  Integrator : Integrator
  R : Gain  Gain=param.R
  Sum : Sum  Inputs=|+-
  Sum1 : Sum  Inputs=|+-
  km 1 : Gain  Gain=param.km
  km 2 : Gain  Gain=param.km
  i (A) : Outport
  tau (Nm) : Outport  Port=2
  wires:
  km 1/1 -> tau (Nm)/1
  km 2/1 -> Sum/2
  omega1 (rad/sec)/1 -> km 2/1
  1/L/1 -> Integrator/1
  Sum/1 -> Sum1/1
  Sum1/1 -> 1/L/1
  u (V)/1 -> Sum/1
  Integrator/1 -> R/1, km 1/1, i (A)/1
  R/1 -> Sum1/2

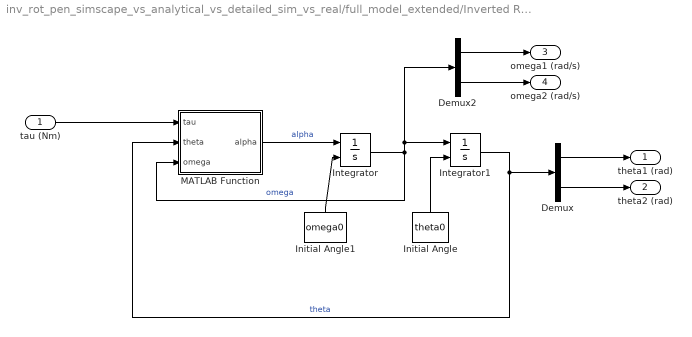
== system inv_rot_pen_simscape_vs_analytical_vs_detailed_sim_vs_real/full_model_extended/Inverted Rotary Pendulum Analytical with friction ==
  tau (Nm) : Inport
  Demux : Demux  Outputs=2
  Demux2 : Demux  Outputs=2
  Initial Angle : Constant  Value=theta0
  Initial Angle1 : Constant  Value=omega0
  Integrator : Integrator  InitialConditionSource=external
  Integrator1 : Integrator  InitialConditionSource=external  InitialCondition=[0.1;0]
  MATLAB Function : MATLAB Function  TreatAsAtomicUnit=on
  theta1 (rad) : Outport
  theta2 (rad) : Outport  Port=2
  omega1 (rad/s) : Outport  Port=3
  omega2 (rad/s) : Outport  Port=4
  wires:
  Initial Angle1/1 -> Integrator/2
  Demux2/2 -> omega2 (rad/s)/1
  Initial Angle/1 -> Integrator1/2
  Demux2/1 -> omega1 (rad/s)/1
  Integrator/1 -> MATLAB Function/3(omega), Integrator1/1, Demux2/1  "omega"
  Demux/1 -> theta1 (rad)/1
  Integrator1/1 -> Demux/1, MATLAB Function/2(theta)  "theta"
  tau (Nm)/1 -> MATLAB Function/1(tau)
  MATLAB Function/1(alpha) -> Integrator/1  "alpha"
  Demux/2 -> theta2 (rad)/1

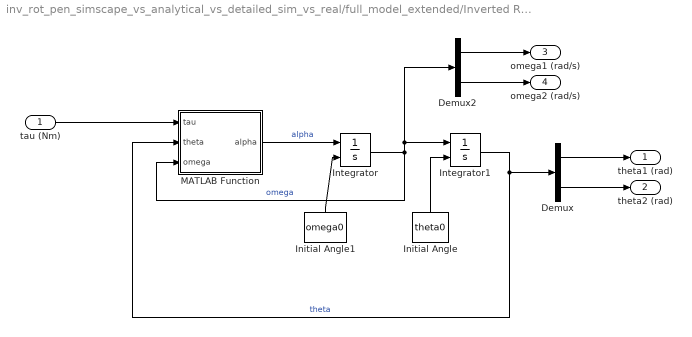
== system inv_rot_pen_simscape_vs_analytical_vs_detailed_sim_vs_real/full_model_extended/Inverted Rotary Pendulum Analytical1 ==
  tau (Nm) : Inport
  Demux : Demux  Outputs=2
  Demux2 : Demux  Outputs=2
  Initial Angle : Constant  Value=theta0
  Initial Angle1 : Constant  Value=omega0
  Integrator : Integrator  InitialConditionSource=external
  Integrator1 : Integrator  InitialConditionSource=external  InitialCondition=[0.1;0]
  MATLAB Function : MATLAB Function  TreatAsAtomicUnit=on
  theta1 (rad) : Outport
  theta2 (rad) : Outport  Port=2
  omega1 (rad/s) : Outport  Port=3
  omega2 (rad/s) : Outport  Port=4
  wires:
  Demux/2 -> theta2 (rad)/1
  MATLAB Function/1(alpha) -> Integrator/1  "alpha"
  tau (Nm)/1 -> MATLAB Function/1(tau)
  Integrator1/1 -> MATLAB Function/2(theta), Demux/1  "theta"
  Demux/1 -> theta1 (rad)/1
  Integrator/1 -> Demux2/1, Integrator1/1, MATLAB Function/3(omega)  "omega"
  Demux2/1 -> omega1 (rad/s)/1
  Initial Angle/1 -> Integrator1/2
  Demux2/2 -> omega2 (rad/s)/1
  Initial Angle1/1 -> Integrator/2
